simulink model "regulator_kf"  (R2019a)
settings: Solver=FixedStepDiscrete  StartTime=0.0  StopTime=50  FixedStep=sT  RelTol=1e-3
InitFcn:
  | param_kf;
values from neighbouring files (symbols this model uses):
  Ad = [1 dt; dt*w^2 1]    [discrete.m]
  Bd = [0; -dt*w^2]    [discrete.m]
  inix = [0.00 0.0]'    [param.m]    (also in param2.m = [0.05 0.0]'; param_kf.m = [0.0 0.0]')
  iniXzmax = 0.07    [param.m]    (also in param2.m; param_kf.m)
  iniXzmin = -0.07    [param.m]    (also in param2.m; param_kf.m)
  K = [k1 k2]    [continus.m]    (also in discrete.m = -place(A, B, [q1 q2]); param.m; param2.m = dlqr(A,B,Q,H); param_kf.m = -place(A, B, [q1 q2]))
  Q = diag([0.1 0.1])    [param2.m]    (also in param_kf.m = 0)
  q2 = -0.00005    (= -5e-05)    [discrete.m]    (also in param.m = -0.6; param2.m = -0.5; param_kf.m = -0.5; test0.m = -8-4j)
  R = 0.001    [param_kf.m]
  sT = 0.01    [discrete.m]    (also in param.m; param2.m; param_kf.m; test0.m)
  w = sqrt(g/zc)    [param_kf.m]    (also in test0.m)
undefined symbols (not defined in the file or in its folder): Cd, Dd, Discrete, Time
libraries: simulink x1, ctrlSharedLib x1
settings Model: Creator=hideaki  LastModifiedBy=hideaki

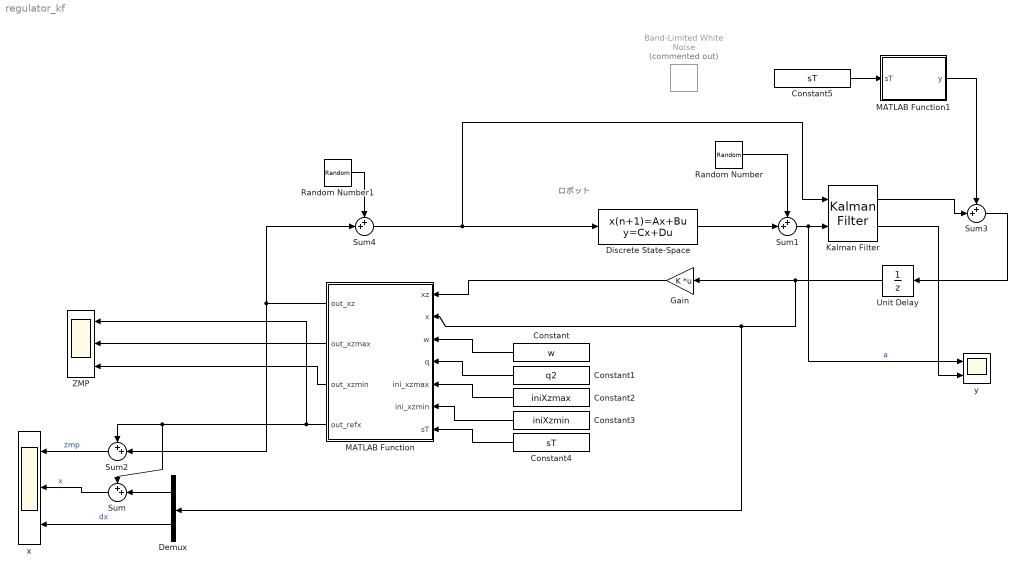
== system regulator_kf ==
  note: ロボット
  Band-Limited White Noise : simulink/Sources/Band-Limited White Noise  Commented=on  Cov=[0.0001]  Ts=sT  seed=[23341]
  Constant : Constant  Value=w
  Constant1 : Constant  Value=q2
  Constant2 : Constant  Value=iniXzmax
  Constant3 : Constant  Value=iniXzmin
  Constant4 : Constant  Value=sT
  Constant5 : Constant  Value=sT
  Demux : Demux  Outputs=2
  Discrete State-Space : DiscreteStateSpace  A=Ad  B=Bd  C=Cd  D=Dd  InitialCondition=inix  SampleTime=sT
  Gain : Gain  Gain=K  Multiplication=Matrix(K*u)
  Kalman Filter : ctrlSharedLib/Kalman Filter  TimeDomain=Discrete-Time  UseCurrentEstimator=on  ModelSource=Individual A, B, C, D matrices  ModelSourceVariable=ss(0.95,1,1,0,1)  A=Ad  B=Bd  C=Cd  D=Dd  NumberOfStates=1  NumberOfInputs=1  NumberOfOutputs=1  InitialEstimateSource=Dialog  X0=inix  P0=10  UseK=off  UseGH=off  NumberOfProcessNoiseInputs=1  G=[0 0]'  TimeInvariantG=on  H=10  TimeInvariantH=on  Q=Q  TimeInvariantQ=on  R=R  TimeInvariantR=on  N=0  TimeInvariantN=on  AddInputPort=on  AddEnablePort=off  OutputEstimatedY=on  OutputP=off  Ts=sT
      settings: SourceProductBaseCode=CT
  MATLAB Function : MATLAB Function  TreatAsAtomicUnit=on  SystemSampleTime=sT
  MATLAB Function1 : MATLAB Function  TreatAsAtomicUnit=on
  Random Number : RandomNumber  Variance=R  SampleTime=sT
  Random Number1 : RandomNumber  Variance=Q  SampleTime=sT
  Sum{,1..4} (5 alike) : Sum  Inputs=++|
  Unit Delay : UnitDelay  SampleTime=-1  HasFrameUpgradeWarning=on
  ZMP : Scope  NumInputPorts=3
  x : Scope  NumInputPorts=3
  y : Scope  NumInputPorts=2
  wires:
  Constant5/1 -> MATLAB Function1/1(sT)
  Demux/1 -> Sum/2
  Sum2/1 -> x/1  "zmp"
  Demux/2 -> x/3  "dx"
  MATLAB Function/3(out_xzmin) -> ZMP/3
  Sum/1 -> x/2  "x"
  MATLAB Function/4(out_refx) -> Sum2/1, Sum/1, ZMP/1
  Constant4/1 -> MATLAB Function/7(sT)
  MATLAB Function/2(out_xzmax) -> ZMP/2
  Constant/1 -> MATLAB Function/3(w)
  Gain/1 -> MATLAB Function/1(xz)
  Constant2/1 -> MATLAB Function/5(ini_xzmax)
  MATLAB Function/1(out_xz) -> Sum2/2, Sum4/2
  Constant3/1 -> MATLAB Function/6(ini_xzmin)
  Constant1/1 -> MATLAB Function/4(q)
  MATLAB Function1/1(y) -> Sum3/1
  Unit Delay/1 -> MATLAB Function/2(x), Demux/1, Gain/1
  Kalman Filter/1 -> Sum3/2
  Sum3/1 -> Unit Delay/1
  Sum1/1 -> y/1, Kalman Filter/2  "a"
  Discrete State-Space/1 -> Sum1/2
  Sum4/1 -> Kalman Filter/1, Discrete State-Space/1
  Random Number/1 -> Sum1/1
  Kalman Filter/2 -> y/2
  Random Number1/1 -> Sum4/1

== matlab function regulator_kf/MATLAB Function1 ==
  data: y output; sT input
function y = nois(sT)
    
    y = zeros(2,1);
    persistent tCnt;
    if isempty(tCnt)
        tCnt = 0;
    end
    
    if (tCnt >= 1 && tCnt <= 1.06) 
        y(2) = -0.2;
    end
    
    tCnt = tCnt + sT;
end

== matlab function regulator_kf/MATLAB Function ==
  data: xz input; out_xz output; x input; out_xzmax output; out_xzmin output; w input; q input; ini_xzmax input; ini_xzmin input; sT input; out_refx output
%%
% ZMPの出力
% 
%
function [out_xz,out_xzmax,out_xzmin,out_refx] = fcn(xz,x,w,q,ini_xzmax,ini_xzmin,sT)
    
    persistent tCnt;
    
    %重心の参照位置（目標値）
    persistent refx;
    %実際の支持領域
    persistent xzmax;
    persistent xzmin;
    %refxを基準にした支持領域
    persistent Xzmax;
    persistent Xzmin;
    
    %以下、離床時に計算されて、着地まで保持した後に着地で出力
    persistent s_xz;
    persistent landing;
    persistent s_xzmax;
    persistent s_xzmin;
    persistent s_refx;
    
    %refxを基準にした重心の位置
    X = 0;
    %refxを基準にした重心の速度（速度はどこを基準にしても変わらない）
    dX = 0;
    %refxを基準にしたZMP
    Xz = 0;
    
    if isempty(tCnt)
        tCnt = 0;
        xzmax = ini_xzmax;
        xzmin = ini_xzmin;
        s_xz = xz;
        landing = 0;
        s_xzmax = xzmax;
        s_xzmin = xzmin;
        s_refx = 0;
        refx = getRefx(xzmax,xzmin);
        Xzmax = xzmax - refx;
        Xzmin = xzmin - refx;
    end
    
    X = x(1) - refx;
    dX = x(2);
    Xz = xz -refx;
    
    %立位化安定領域から外れた（xzmin以下）
    if (X+(dX/w) <= Xzmin) 
        %両足支持
        %支持領域を広げるために、まずは片足支持に移行する
        if (xzmax == 0.07 && xzmin == -0.07 && landing == 0)
            %強制的に支持領域を狭める（傾いてる方の足を上げる）
            xzmin = 0.01;
            refx = getRefx(xzmax,xzmin);
            %実際のZMP
            s_xz = Xz +refx; 
            %両足支持の場合は離床なのですぐに反映する
            xz = s_xz;
            
            %重心の参照位置は、この時点では変えない
            refx = 0;
            
            %refxを基準としたZMP
            Xz = (1-q)*(X+(dX/w));
            Xzmin = Xz;
            s_xzmin = Xzmin + refx;
            s_refx = getRefx(xzmax,s_xzmin);
            %実際のZMP（片足支持の場合は着地までに0.6秒かかる）
            s_xz = Xz + refx;
            %着地まで待ち
            tCnt = 0;
            landing = 1;
        end
    end
    
    %着地
    if (tCnt >= 0.6 && landing == 1) 
        xzmin = s_xzmin;
        refx = s_refx;
        xz = s_xz;
        landing = 2;
    elseif (landing == 1)
        %実際のロボットでは、ここで両足の中心を重心の参照位置にする（ロボットの遊脚は毎時刻動いている）
        %refx = refx - (abs(s_xzmin) + abs(xzmax))/0.6;
        
    end
    
    %{
    %立位化安定領域から外れた（xzmin以下）
    if (X+(dX/w) <= Xzmin) 
        %両足支持
        %支持領域を広げるために、まずは片足支持に移行する
        if (xzmax == 0.07 && xzmin == -0.07)
            %強制的に支持領域を狭める（傾いてる方の足を上げる）
            xzmin = 0.01;
            refx = getRefx(xzmax,xzmin);
            %実際のZMP
            s_xz = Xz +refx; 
            %両足支持の場合は離床なのですぐに反映する
            xz = s_xz;
            landing = 0;
        %片足支持
        elseif (landing == 0)
                
            %refxを基準としたZMP
            Xz = (1-q)*(X+(dX/w));
            Xzmin = Xz;
            s_xzmin = Xzmin + refx;
            s_refx = getRefx(xzmax,xzmin);
            %実際のZMP（片足支持の場合は着地までに0.6秒かかる）
            s_xz = Xz + refx;
            %着地まで待ち
            tCnt = 0;
            landing = 1;
        end
    end
    
    if (tCnt >= 0.6 && landing == 1) 
        xzmin = s_xzmin;
        refx = s_refx;
        xz = s_xz;
        landing = 2;
    end
    %}
            
    %{
    %着地まで0.6秒と仮定(歩行パターンの1歩にかかる秒数）
    if (tCnt >= 0.6) 
        %立位化安定領域から外れた（xzmin以下）
        if (X+(dX/w) <= Xzmin) 
            
            %両足支持
            %支持領域を広げるために、まずは片足支持に移行する
            if (xzmax == 0.07 && xzmin == -0.07)
                %強制的に支持領域を狭める（傾いてる方の足を上げる）
                xzmin = 0.01;
                refx = getRefx(xzmax,xzmin);
                %実際のZMP
                xz = Xz +refx; 
                
                %着地まで待ち
                tCnt = 0;
            
            %片足支持
            else
                %refxを基準としたZMP
                Xz = (1-q)*(X+(dX/w));
                Xzmin = Xz;
                xzmin = Xzmin + refx;
                refx = getRefx(xzmax,xzmin);
                %実際のZMP
                xz = Xz + refx;
            end
        end
        %立位化安定領域から外れた（xzmax以上）
        if (X+(dX/w) >= xzmax)
            
        end
    end
    %}
    
    %支持領域の拘束
    if (xz > xzmax) 
        out_xz = xzmax;      
    elseif (xz < xzmin)
        out_xz = xzmin;   
    else
        out_xz = xz;
    end
    
    out_xzmax = xzmax;
    out_xzmin = xzmin;
    out_refx = refx;
    
    tCnt = tCnt + sT;
end

%%
% 重心の参照位置
%
function refx = getRefx(xzmax,xzmin) 
    
    if (0 > xzmax)
        refx = xzmax;
    elseif (0 < xzmin) 
        refx = xzmin;
    else
        refx = (xzmax+xzmin)/2;
    end
    
end
